simulink model "velocity_control"  (R2018a)
settings: Solver=VariableStepAuto  StartTime=0.0  StopTime=20  RelTol=1e-3
undefined symbols (not defined in the file): sigbuilder_block
settings Model: Creator=BEAR  LastModifiedBy=BEAR

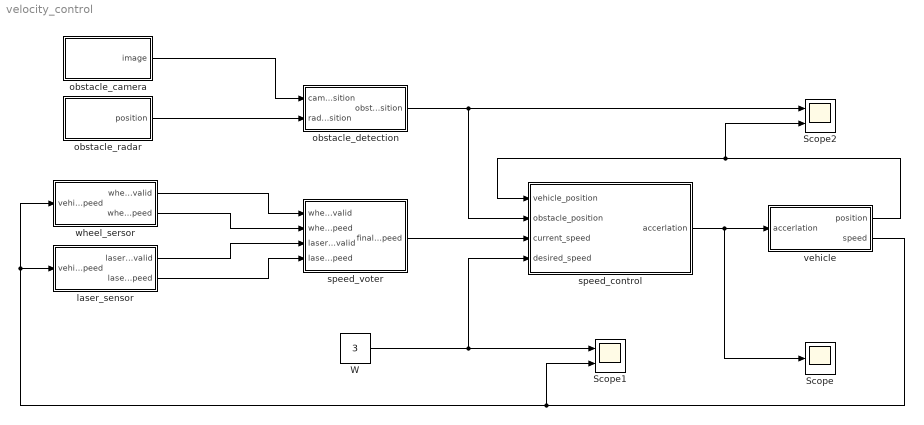
== system velocity_control ==
  Scope : Scope
  Scope1 : Scope  NumInputPorts=2
  Scope2 : Scope  NumInputPorts=2
  W : Constant  Value=3
  laser_sensor : Subsystem
  obstacle_camera : Subsystem  Tag=STV Subsys  LoadFcn=sigbuilder_block('load');  StartFcn=sigbuilder_block('start');  StopFcn=sigbuilder_block('stop');  ClipboardFcn=sigbuilder_block('clipboard');  mask(Sigbuilder block){tuvar=[0:10]}
      mask help: Simulink:masks:SigbuilderBlock_MD
      mask init:
      | if ~strcmp(get_param(bdroot(gcbh),'SimulationStatus'),'stopped') tuvar = sigbuilder_block('maskInit'); end
      settings: CopyFcn=sigbuilder_block('copy');  DeleteFcn=sigbuilder_block('delete');  ModelCloseFcn=sigbuilder_block('modelClose');  PreSaveFcn=sigbuilder_block('preSave');  PauseFcn=sigbuilder_block('pause');  ContinueFcn=sigbuilder_block('continue');  NameChangeFcn=sigbuilder_block('namechange');  OpenFcn=sigbuilder_block('open',[0 68 1280 636 ]);  CloseFcn=sigbuilder_block('close');
      mask Display: plot(0, 0, 100, 100,[2, 2, 32, 32, 2], [68, 8, 8, 68, 68],[32, 2], [38, 38], [32, 19, 2],[53, 60, 44], [32, 17, 17, 2],[16, 16, 31, 31]);txt = getActiveGroup(gcbh);text(2, 100, txt,'verticalAlignment', 'top');
  obstacle_detection : Subsystem
  obstacle_radar : Subsystem  Tag=STV Subsys  LoadFcn=sigbuilder_block('load');  StartFcn=sigbuilder_block('start');  StopFcn=sigbuilder_block('stop');  ClipboardFcn=sigbuilder_block('clipboard');  mask(Sigbuilder block){tuvar=[0:10]}
      mask help: Simulink:masks:SigbuilderBlock_MD
      mask init:
      | if ~strcmp(get_param(bdroot(gcbh),'SimulationStatus'),'stopped') tuvar = sigbuilder_block('maskInit'); end
      settings: CopyFcn=sigbuilder_block('copy');  DeleteFcn=sigbuilder_block('delete');  ModelCloseFcn=sigbuilder_block('modelClose');  PreSaveFcn=sigbuilder_block('preSave');  PauseFcn=sigbuilder_block('pause');  ContinueFcn=sigbuilder_block('continue');  NameChangeFcn=sigbuilder_block('namechange');  OpenFcn=sigbuilder_block('open',[0 68 1280 636 ]);  CloseFcn=sigbuilder_block('close');
      mask Display: plot(0, 0, 100, 100,[2, 2, 32, 32, 2], [68, 8, 8, 68, 68],[32, 2], [38, 38], [32, 19, 2],[53, 60, 44], [32, 17, 17, 2],[16, 16, 31, 31]);txt = getActiveGroup(gcbh);text(2, 100, txt,'verticalAlignment', 'top');
  speed_control : Subsystem
  speed_voter : Subsystem
  vehicle : Subsystem
  wheel_sersor : Subsystem
  wires:
  obstacle_camera/1(image) -> obstacle_detection/1(camera_position)
  wheel_sersor/2(wheel_speed) -> speed_voter/2(wheel_speed)
  laser_sensor/1(laser_valid) -> speed_voter/3(laser_valid)
  wheel_sersor/1(wheel_valid) -> speed_voter/1(wheel_valid)
  laser_sensor/2(laser_speed) -> speed_voter/4(laser_speed)
  speed_voter/1(final_speed) -> speed_control/3(current_speed)
  obstacle_detection/1(obstacle_position) -> speed_control/2(obstacle_position), Scope2/1
  W/1 -> Scope1/1, speed_control/4(desired_speed)
  speed_control/1(accerlation) -> Scope/1, vehicle/1(accerlation)
  vehicle/2(speed) -> Scope1/2, wheel_sersor/1(vehicle_speed), laser_sensor/1(vehicle_speed)
  vehicle/1(position) -> Scope2/2, speed_control/1(vehicle_position)
  obstacle_radar/1(position) -> obstacle_detection/2(radar_position)

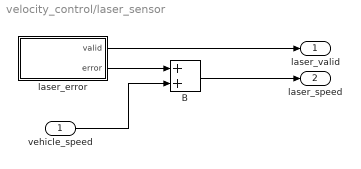
== system velocity_control/laser_sensor ==
  vehicle_speed : Inport
  B : Sum  SampleTime=0.1
  laser_error : Subsystem  Tag=STV Subsys  LoadFcn=sigbuilder_block('load');  StartFcn=sigbuilder_block('start');  StopFcn=sigbuilder_block('stop');  ClipboardFcn=sigbuilder_block('clipboard');  mask(Sigbuilder block){tuvar=[0:10]}
      mask help: Simulink:masks:SigbuilderBlock_MD
      mask init:
      | if ~strcmp(get_param(bdroot(gcbh),'SimulationStatus'),'stopped') tuvar = sigbuilder_block('maskInit'); end
      settings: CopyFcn=sigbuilder_block('copy');  DeleteFcn=sigbuilder_block('delete');  ModelCloseFcn=sigbuilder_block('modelClose');  PreSaveFcn=sigbuilder_block('preSave');  PauseFcn=sigbuilder_block('pause');  ContinueFcn=sigbuilder_block('continue');  NameChangeFcn=sigbuilder_block('namechange');  OpenFcn=sigbuilder_block('open',[0 68 1280 636 ]);  CloseFcn=sigbuilder_block('close');
      mask Display: plot(0, 0, 100, 100,[2, 2, 32, 32, 2], [68, 8, 8, 68, 68],[32, 2], [38, 38], [32, 19, 2],[53, 60, 44], [32, 17, 17, 2],[16, 16, 31, 31]);txt = getActiveGroup(gcbh);text(2, 100, txt,'verticalAlignment', 'top');
  laser_valid : Outport
  laser_speed : Outport  Port=2
  wires:
  laser_error/2(error) -> B/1
  vehicle_speed/1 -> B/2
  laser_error/1(valid) -> laser_valid/1
  B/1 -> laser_speed/1

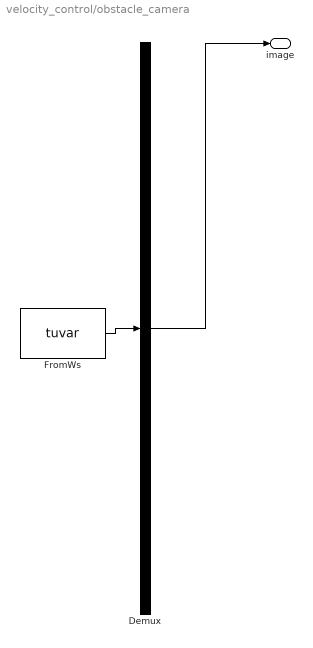
== system velocity_control/obstacle_camera ==
  Demux : Demux  Tag=STV Demux  Outputs=1
  FromWs : FromWorkspace  Tag=STV FromWs  VariableName=tuvar  SampleTime=0
      SigBuilderData=|
      | common.afterFinalStr = 'Extrapolate'
      | common.sampleTime = 0
      | dataSet.timeRange = [0 20]
      | dataSet.name = 'Group 1'
      | sbobj.Groups.Name = 'Group 1'
      | sbobj.Groups.Signals.Name = 'image'
      | sbobj.Groups.Signals.XData = [0 4 6 20]
      | sbobj.Groups.Signals.YData = [-1 -1 -1 -1]
      | sbobj.Groups.TimeRange = [0 20]
  image : Outport  Tag=STV Outport
  wires:
  Demux/1 -> image/1
  FromWs/1 -> Demux/1

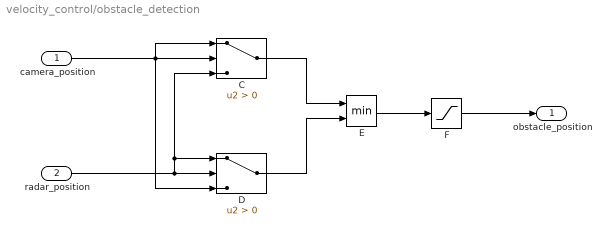
== system velocity_control/obstacle_detection ==
  camera_position : Inport
  radar_position : Inport  Port=2
  C : Switch  Criteria=u2 > Threshold  SampleTime=0.1
  D : Switch  Criteria=u2 > Threshold  SampleTime=0.1
  E : MinMax  Inputs=2  SampleTime=0.1
  F : Saturate  UpperLimit=100  LowerLimit=0  SampleTime=0.1
  obstacle_position : Outport
  wires:
  camera_position/1 -> D/3, C/1, C/2
  radar_position/1 -> D/1, C/3, D/2
  C/1 -> E/1
  D/1 -> E/2
  E/1 -> F/1
  F/1 -> obstacle_position/1

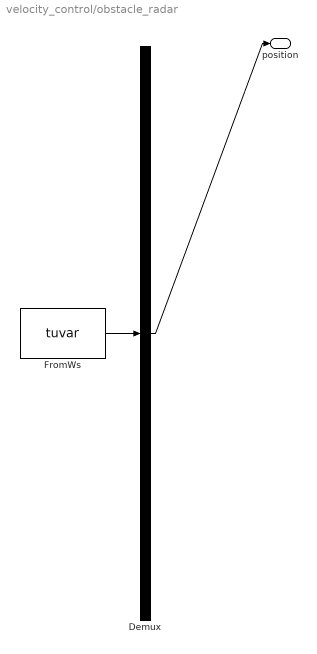
== system velocity_control/obstacle_radar ==
  Demux : Demux  Tag=STV Demux  Outputs=1
  FromWs : FromWorkspace  Tag=STV FromWs  VariableName=tuvar  SampleTime=0
      SigBuilderData=|
      | common.afterFinalStr = 'Extrapolate'
      | common.sampleTime = 0
      | dataSet.timeRange = [0 20]
      | dataSet.name = 'Group 1'
      | sbobj.Groups.Name = 'Group 1'
      | sbobj.Groups.Signals.Name = 'position'
      | sbobj.Groups.Signals.XData = [0 6 6 10 10 14 14 20]
      | sbobj.Groups.Signals.YData = [0 0 25 30 0 0 45 45]
      | sbobj.Groups.TimeRange = [0 20]
  position : Outport  Tag=STV Outport
  wires:
  FromWs/1 -> Demux/1
  Demux/1 -> position/1

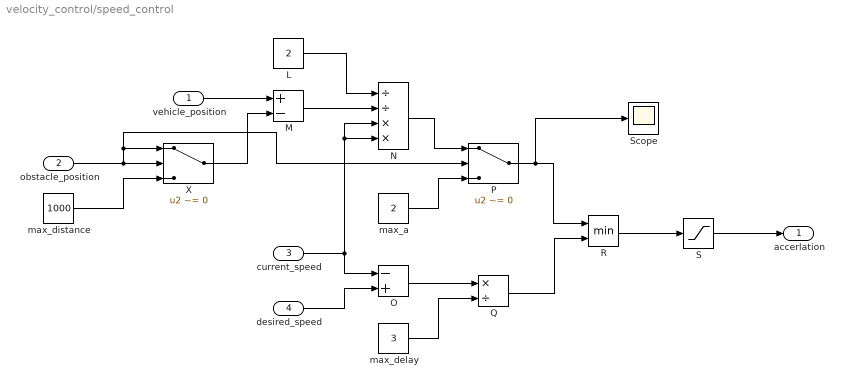
== system velocity_control/speed_control ==
  vehicle_position : Inport
  obstacle_position : Inport  Port=2
  current_speed : Inport  Port=3
  desired_speed : Inport  Port=4
  L : Constant  Value=2
  M : Sum  Inputs=+-  SampleTime=0.1
  N : Product  Inputs=//**  SampleTime=0.1
  O : Sum  Inputs=-+  SampleTime=0.1
  P : Switch  Criteria=u2 ~= 0  SampleTime=0.1
  Q : Product  Inputs=*/  SampleTime=0.1
  R : MinMax  Inputs=2  SampleTime=0.1
  S : Saturate  UpperLimit=2  LowerLimit=-2  SampleTime=0.1
  Scope : Scope
  X : Switch  Criteria=u2 ~= 0  SampleTime=0.1
  max_a : Constant  Value=2
  max_delay : Constant  Value=3
  max_distance : Constant  Value=1000
  accerlation : Outport
  wires:
  current_speed/1 -> N/3, N/4, O/1
  desired_speed/1 -> O/2
  O/1 -> Q/1
  max_delay/1 -> Q/2
  L/1 -> N/1
  R/1 -> S/1
  S/1 -> accerlation/1
  N/1 -> P/1
  max_a/1 -> P/3
  P/1 -> Scope/1, R/1
  Q/1 -> R/2
  M/1 -> N/2
  vehicle_position/1 -> M/1
  obstacle_position/1 -> P/2, X/1, X/2
  max_distance/1 -> X/3
  X/1 -> M/2

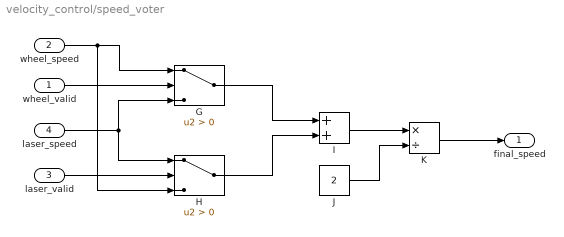
== system velocity_control/speed_voter ==
  wheel_valid : Inport
  wheel_speed : Inport  Port=2
  laser_valid : Inport  Port=3
  laser_speed : Inport  Port=4
  G : Switch  Criteria=u2 > Threshold  SampleTime=0.1
  H : Switch  Criteria=u2 > Threshold  SampleTime=0.1
  I : Sum  SampleTime=0.1
  J : Constant  Value=2
  K : Product  Inputs=*/  SampleTime=0.1
  final_speed : Outport
  wires:
  wheel_valid/1 -> G/2
  wheel_speed/1 -> H/3, G/1
  laser_speed/1 -> H/1, G/3
  laser_valid/1 -> H/2
  G/1 -> I/1
  H/1 -> I/2
  I/1 -> K/1
  K/1 -> final_speed/1
  J/1 -> K/2

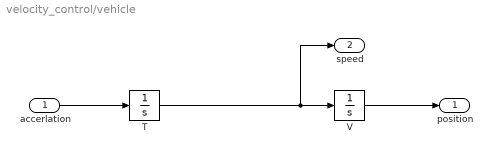
== system velocity_control/vehicle ==
  accerlation : Inport
  T : Integrator
  V : Integrator
  position : Outport
  speed : Outport  Port=2
  wires:
  accerlation/1 -> T/1
  T/1 -> speed/1, V/1
  V/1 -> position/1

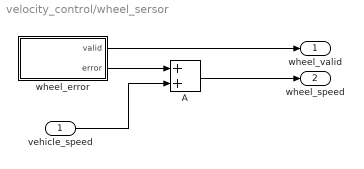
== system velocity_control/wheel_sersor ==
  vehicle_speed : Inport
  A : Sum  SampleTime=0.1
  wheel_error : Subsystem  Tag=STV Subsys  LoadFcn=sigbuilder_block('load');  StartFcn=sigbuilder_block('start');  StopFcn=sigbuilder_block('stop');  ClipboardFcn=sigbuilder_block('clipboard');  mask(Sigbuilder block){tuvar=[0:10]}
      mask help: Simulink:masks:SigbuilderBlock_MD
      mask init:
      | if ~strcmp(get_param(bdroot(gcbh),'SimulationStatus'),'stopped') tuvar = sigbuilder_block('maskInit'); end
      settings: CopyFcn=sigbuilder_block('copy');  DeleteFcn=sigbuilder_block('delete');  ModelCloseFcn=sigbuilder_block('modelClose');  PreSaveFcn=sigbuilder_block('preSave');  PauseFcn=sigbuilder_block('pause');  ContinueFcn=sigbuilder_block('continue');  NameChangeFcn=sigbuilder_block('namechange');  OpenFcn=sigbuilder_block('open',[0 68 1280 636 ]);  CloseFcn=sigbuilder_block('close');
      mask Display: plot(0, 0, 100, 100,[2, 2, 32, 32, 2], [68, 8, 8, 68, 68],[32, 2], [38, 38], [32, 19, 2],[53, 60, 44], [32, 17, 17, 2],[16, 16, 31, 31]);txt = getActiveGroup(gcbh);text(2, 100, txt,'verticalAlignment', 'top');
  wheel_valid : Outport
  wheel_speed : Outport  Port=2
  wires:
  wheel_error/2(error) -> A/1
  vehicle_speed/1 -> A/2
  wheel_error/1(valid) -> wheel_valid/1
  A/1 -> wheel_speed/1

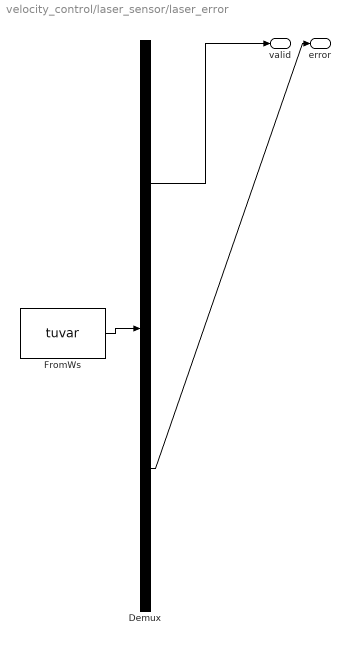
== system velocity_control/laser_sensor/laser_error ==
  Demux : Demux  Tag=STV Demux  Outputs=2
  FromWs : FromWorkspace  Tag=STV FromWs  VariableName=tuvar  SampleTime=0
      SigBuilderData=|
      | common.afterFinalStr = 'Extrapolate'
      | common.sampleTime = 0
      | dataSet.timeRange = [0 20]
      | dataSet.name = 'Group 1'
      | sbobj.Groups.Name = 'Group 1'
      | sbobj.Groups.Signals(1).Name = 'valid'
      | sbobj.Groups.Signals(1).XData = [0 4 6 20]
      | sbobj.Groups.Signals(1).YData = [1 1 1 1]
      | sbobj.Groups.Signals(2).Name = 'error'
      | sbobj.Groups.Signals(2).XData = [0 0.14 0.14 0.26 0.26 0.38 0.38 0.46 0.46 0.6 0.6 0.72 0.72 0.86 0.86 1 1 1.28 1.28 1.64 1.64 2 2 2.3 2.3 2.62 2.62 3 3 3.48 3.48 4 4 4.48 4.48 5 5 5.46 5.46 6 6 6.48 6.48 7 7 7.46 7.46 8 8 8.48 8.48 9 9 9.58 9.58 10 10 20]
      | sbobj.Groups.Signals(2).YData = [0.07 0.07 0.028 0.028 -0.036 -0.036 0.1 0.1 -0.02 -0.02 0.1 0.1 -0.038 -0.038 0.068 0.068 -0.024 -0.024 0.024 0.024 0.06 0.06 -0.014 -0.014 0.082 0.082 -0.032 -0.032 -0.01 -0.01 -0.072 -0.072 0.068 0.068 0.032 0.032 -0.084 -0.084 0.084 0.084 0.06 0.06 0.022 0.022 -0.034 -0.034 0.038 0.038 -0.074 -0.074 0.062 0.062 -0.028 -0.028 0.018 0.018 0 0]
      | sbobj.Groups.TimeRange = [0 20]
  valid : Outport  Tag=STV Outport
  error : Outport  Tag=STV Outport  Port=2
  wires:
  Demux/1 -> valid/1
  FromWs/1 -> Demux/1
  Demux/2 -> error/1

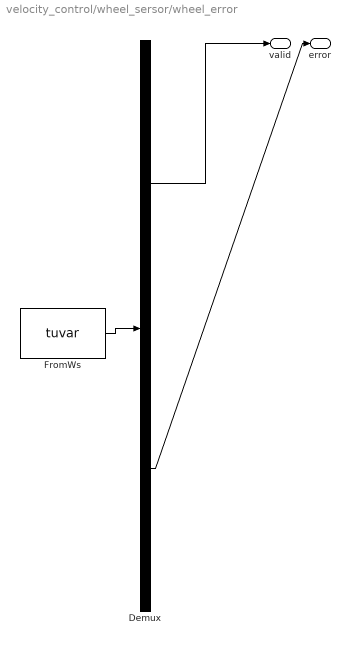
== system velocity_control/wheel_sersor/wheel_error ==
  Demux : Demux  Tag=STV Demux  Outputs=2
  FromWs : FromWorkspace  Tag=STV FromWs  VariableName=tuvar  SampleTime=0
      SigBuilderData=|
      | common.afterFinalStr = 'Extrapolate'
      | common.sampleTime = 0
      | dataSet.timeRange = [0 20]
      | dataSet.name = 'Group 1'
      | sbobj.Groups.Name = 'Group 1'
      | sbobj.Groups.Signals(1).Name = 'valid'
      | sbobj.Groups.Signals(1).XData = [0 4 6 20]
      | sbobj.Groups.Signals(1).YData = [-1 -1 -1 -1]
      | sbobj.Groups.Signals(2).Name = 'error'
      | sbobj.Groups.Signals(2).XData = [0 20]
      | sbobj.Groups.Signals(2).YData = [0 0]
      | sbobj.Groups.TimeRange = [0 20]
  valid : Outport  Tag=STV Outport
  error : Outport  Tag=STV Outport  Port=2
  wires:
  Demux/1 -> valid/1
  FromWs/1 -> Demux/1
  Demux/2 -> error/1
